simulink model "ieee_6_bus_base_case_hydro_dominated"  (R2015b)
settings: Solver=ode23t  StartTime=0.0  StopTime=25  FixedStep=Ts  RelTol=1e-3
values from neighbouring files (symbols this model uses):
  Cbase = 1/(100*pi*Xbase)    (= 1.34217357979e-05)    [ieee_6_bus.m]
  Lbase = Xbase/(100*pi)    (= 0.754903726073)    [ieee_6_bus.m]
  Ts = 1e-5    (= 1e-05)    [ieee_6_bus.m]
  Xbase = (Vbase^2)/Sbase    (= 237.16)    [ieee_6_bus.m]
undefined symbols (not defined in the file or in its folder): loadconnection, startup
libraries: powerlib x170, powerlib_meascontrol x15, simulink x10, sps_avr x4, powerlib_extras x1
(part 2 of 3)

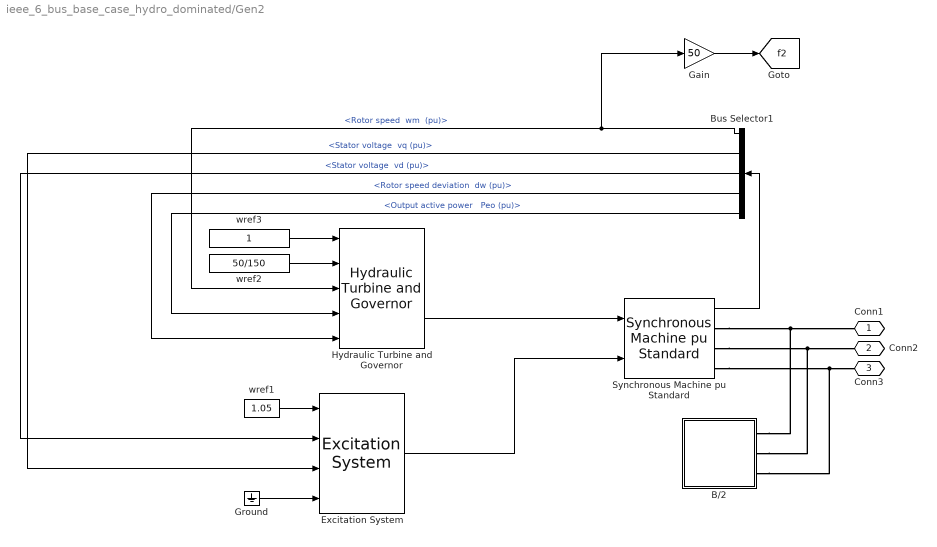
== system ieee_6_bus_base_case_hydro_dominated/Gen2 ==
  B/2 : Subsystem
  Bus Selector1 : BusSelector  OutputSignals="Mechanical.Rotor speed  wm  (pu),dq0 components.Stator voltage  vq (pu),dq0 components.Stator voltage  vd (pu),Mechanical.Rotor speed deviation  dw (pu),Output active power   Peo (pu)"
  Excitation System : sps_avr/Excitation System  tr=20e-3  reg=[ 350, 0.001 ]  exc=[ 1, 0 ]  tgr=[ 0, 0 ]  damp=[ 0.001, 0.1 ]  sat=[ 0, 0 ]  lim=[ -11.5, 11.5, 0 ]  v0="[1.0  1.28]"
  Gain : Gain  Gain=50
  Ground : Ground
  Hydraulic Turbine and Governor : powerlib/Machines/Hydraulic Turbine and Governor  sm="[ 10/3  0.07 ]"  gate="[  0.01  0.97518  -0.1  0.1 ]"  reg="[  0.05  1.163  0.105  0  0.01  ]"  hyd="[  0  2.67  ]"  dref=0  po=1/3
  Synchronous Machine pu Standard : powerlib/Machines/Synchronous Machine pu Standard  PresetModel=No  MechanicalLoad=Mechanical power Pm  ShowDetailedParameters=on  RotorType=Round  Units=per unit standard parameters  MeasurementBus=off  NominalParameters=[150e+06 690 50]  Reactances1=[ 1.81, 0.3, 0.23, 1.76, 0.65, 0.25, 0.15 ]  Reactances2=[2.24 0.17 0.12 1.02 0.13 0.08]  dAxisTimeConstants=Short-circuit  qAxisTimeConstants=Short-circuit  TimeConstants1="[ 4.4849  0.0681  0.1  ]"  TimeConstants2=[ 8.0, 0.03, 1.0, 0.07 ]  TimeConstants3="[  4.49  0.0681  0.0513  ]"  TimeConstants4=[ 8.0, 0.03, 0.3371, 0.0295 ]  TimeConstants5=[ 1.01, 0.053, 0.1 ]  TimeConstants6=[ 1.3201, 0.023, 1.0, 0.07 ]  TimeConstants7=[0.012 0.003 0.003]  TimeConstants8=[ 1.3201, 0.0231, 0.3371, 0.0295 ]  StatorResistance=0.00000107875  Mechanical=[4 0.02056 4]  PolePairs=20  InitialConditions="[ 0  0  0  0  0  0  0  0  1 ]"  SetSaturation=off  Saturation=[0.6404,0.7127,0.8441,0.9214,0.9956,1.082,1.19,1.316,1.457;0.7,0.7698,0.8872,0.9466,0.9969,1.046,1.1,1.151,1.201]  LoadFlowParameters=[1,0,0,0,0]  TsPowergui=0  TsBlock=-1  IterativeModel=Trapezoidal non iterative  BusType=PV  Pref=50e6  Qref=0  Qmin=-inf  Qmax=inf  PLF=0  QLF=0
  wref1 : Constant  Value=1.05
  wref2 : Constant  Value=50/150
  wref3 : Constant
  Conn1 : PMIOPort  Port=1  Side=Right
  Conn2 : PMIOPort  Port=2  Side=Right
  Conn3 : PMIOPort  Port=3  Side=Right
  tag scope: f2=global
  wires:
  Hydraulic Turbine and Governor/2 -> Synchronous Machine pu Standard/1
  Gain/1 -> [f2]
  Bus Selector1/2 -> Excitation System/3  "<Stator voltage  vq (pu)>"
  Bus Selector1/1 -> Hydraulic Turbine and Governor/3, Gain/1  "<Rotor speed  wm  (pu)>"
  Bus Selector1/3 -> Excitation System/2  "<Stator voltage  vd (pu)>"
  Excitation System/1 -> Synchronous Machine pu Standard/2
  Ground/1 -> Excitation System/4
  wref1/1 -> Excitation System/1
  Synchronous Machine pu Standard/1 -> Bus Selector1/1
  wref3/1 -> Hydraulic Turbine and Governor/1
  Bus Selector1/4 -> Hydraulic Turbine and Governor/5  "<Rotor speed deviation  dw (pu)>"
  Bus Selector1/5 -> Hydraulic Turbine and Governor/4  "<Output active power   Peo (pu)>"
  wref2/1 -> Hydraulic Turbine and Governor/2
  connections:
  Synchronous Machine pu Standard/RConn1 -- Conn1/RConn1 -- B/2/RConn1
  Synchronous Machine pu Standard/RConn2 -- Conn2/RConn1 -- B/2/RConn2
  Synchronous Machine pu Standard/RConn3 -- Conn3/RConn1 -- B/2/RConn3

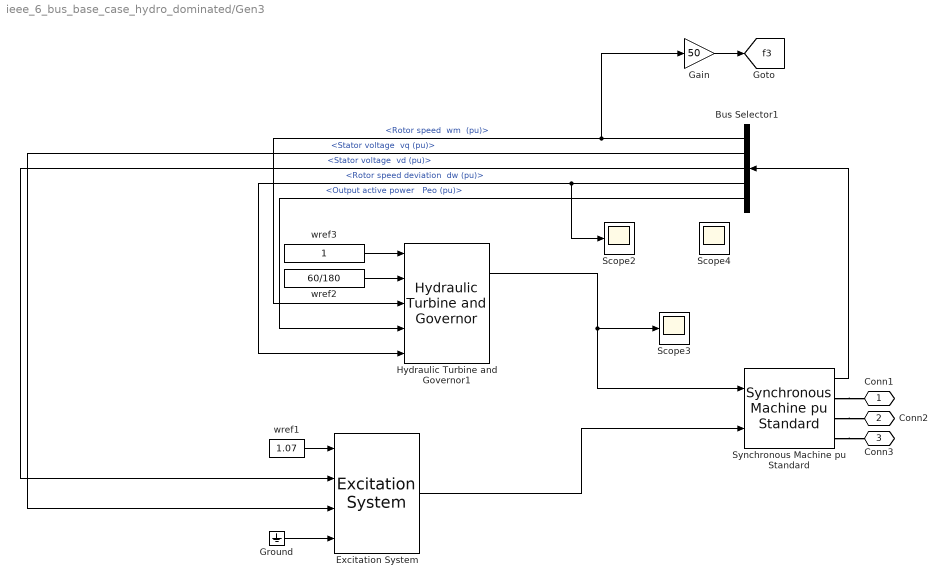
== system ieee_6_bus_base_case_hydro_dominated/Gen3 ==
  Bus Selector1 : BusSelector  OutputSignals="Mechanical.Rotor speed  wm  (pu),dq0 components.Stator voltage  vq (pu),dq0 components.Stator voltage  vd (pu),Mechanical.Rotor speed deviation  dw (pu),Output active power   Peo (pu)"
  Excitation System : sps_avr/Excitation System  tr=20e-3  reg=[ 350, 0.001 ]  exc=[ 1, 0 ]  tgr=[ 0, 0 ]  damp=[ 0.001, 0.1 ]  sat=[ 0, 0 ]  lim=[ -11.5, 11.5, 0 ]  v0="[1.0  1.28]"
  Gain : Gain  Gain=50
  Ground : Ground
  Hydraulic Turbine and Governor1 : powerlib/Machines/Hydraulic Turbine and Governor  sm="[ 10/3  0.07 ]"  gate="[  0.01  0.97518  -0.1  0.1 ]"  reg="[  0.05  1.163  0.105  0  0.01  ]"  hyd="[  0  2.67  ]"  dref=0  po=1/3
  Scope2 : Scope
  Scope3 : Scope
  Scope4 : Scope
  Synchronous Machine pu Standard : powerlib/Machines/Synchronous Machine pu Standard  PresetModel=No  MechanicalLoad=Mechanical power Pm  ShowDetailedParameters=on  RotorType=Round  Units=per unit standard parameters  MeasurementBus=off  NominalParameters=[180e+06 690 50]  Reactances1=[ 1.81, 0.3, 0.23, 1.76, 0.65, 0.25, 0.15 ]  Reactances2=[2.24 0.17 0.12 1.02 0.13 0.08]  dAxisTimeConstants=Short-circuit  qAxisTimeConstants=Short-circuit  TimeConstants1="[ 4.4849  0.0681  0.1  ]"  TimeConstants2=[ 8.0, 0.03, 1.0, 0.07 ]  TimeConstants3="[  4.49  0.0681  0.0513  ]"  TimeConstants4=[ 8.0, 0.03, 0.3371, 0.0295 ]  TimeConstants5=[ 1.01, 0.053, 0.1 ]  TimeConstants6=[ 1.3201, 0.023, 1.0, 0.07 ]  TimeConstants7=[0.012 0.003 0.003]  TimeConstants8=[ 1.3201, 0.0231, 0.3371, 0.0295 ]  StatorResistance=0.00000107875  Mechanical=[4 0.02056 4]  PolePairs=20  InitialConditions="[ 0  0  0  0  0  0  0  0  1 ]"  SetSaturation=off  Saturation=[0.6404,0.7127,0.8441,0.9214,0.9956,1.082,1.19,1.316,1.457;0.7,0.7698,0.8872,0.9466,0.9969,1.046,1.1,1.151,1.201]  LoadFlowParameters=[1,0,0,0,0]  TsPowergui=0  TsBlock=-1  IterativeModel=Trapezoidal non iterative  BusType=PV  Pref=60e6  Qref=0  Qmin=-inf  Qmax=inf  PLF=0  QLF=0
  wref1 : Constant  Value=1.07
  wref2 : Constant  Value=60/180
  wref3 : Constant
  Conn1 : PMIOPort  Port=1  Side=Right
  Conn2 : PMIOPort  Port=2  Side=Right
  Conn3 : PMIOPort  Port=3  Side=Right
  tag scope: f3=global
  wires:
  Synchronous Machine pu Standard/1 -> Bus Selector1/1
  wref1/1 -> Excitation System/1
  Ground/1 -> Excitation System/4
  Excitation System/1 -> Synchronous Machine pu Standard/2
  Bus Selector1/3 -> Excitation System/2  "<Stator voltage  vd (pu)>"
  Bus Selector1/1 -> Hydraulic Turbine and Governor1/3, Gain/1  "<Rotor speed  wm  (pu)>"
  Bus Selector1/2 -> Excitation System/3  "<Stator voltage  vq (pu)>"
  Gain/1 -> [f3]
  Hydraulic Turbine and Governor1/1 -> Synchronous Machine pu Standard/1, Scope3/1
  wref2/1 -> Hydraulic Turbine and Governor1/2
  wref3/1 -> Hydraulic Turbine and Governor1/1
  Bus Selector1/4 -> Hydraulic Turbine and Governor1/5, Scope2/1  "<Rotor speed deviation  dw (pu)>"
  Bus Selector1/5 -> Hydraulic Turbine and Governor1/4  "<Output active power   Peo (pu)>"
  connections:
  Synchronous Machine pu Standard/RConn3 -- Conn3/RConn1
  Synchronous Machine pu Standard/RConn2 -- Conn2/RConn1
  Synchronous Machine pu Standard/RConn1 -- Conn1/RConn1

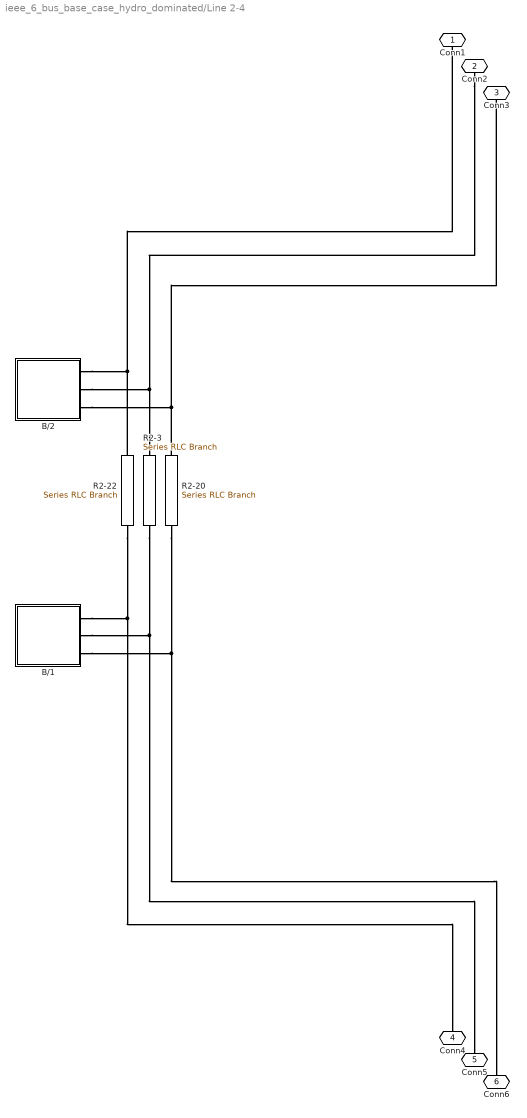
== system ieee_6_bus_base_case_hydro_dominated/Line 2-4 ==
  B/1 : Subsystem
  B/2 : Subsystem
  R2-20 : powerlib/Elements/Series RLC Branch  LConnTagsString=__new0  RConnTagsString=__new0  BranchType=RL  Resistance=0.05*Xbase  Inductance=0.1*Lbase  SetiL0=off  InitialCurrent=0  Capacitance=1e-6  Setx0=off  InitialVoltage=0  Measurements=None
  R2-22 : powerlib/Elements/Series RLC Branch  LConnTagsString=__new0  RConnTagsString=__new0  BranchType=RL  Resistance=0.05*Xbase  Inductance=0.1*Lbase  SetiL0=off  InitialCurrent=0  Capacitance=1e-6  Setx0=off  InitialVoltage=0  Measurements=None
  R2-3 : powerlib/Elements/Series RLC Branch  LConnTagsString=__new0  RConnTagsString=__new0  BranchType=RL  Resistance=0.05*Xbase  Inductance=0.1*Lbase  SetiL0=off  InitialCurrent=0  Capacitance=1e-6  Setx0=off  InitialVoltage=0  Measurements=None
  Conn1 : PMIOPort  Port=1  Side=Right
  Conn2 : PMIOPort  Port=2  Side=Right
  Conn3 : PMIOPort  Port=3  Side=Right
  Conn4 : PMIOPort  Port=4  Side=Left
  Conn5 : PMIOPort  Port=5  Side=Left
  Conn6 : PMIOPort  Port=6  Side=Left
  connections:
  R2-22/RConn1 -- B/1/RConn1 -- Conn4/RConn1
  R2-20/RConn1 -- B/1/RConn3 -- Conn6/RConn1
  Conn2/RConn1 -- B/2/RConn2 -- R2-3/LConn1
  R2-22/LConn1 -- B/2/RConn1 -- Conn1/RConn1
  R2-20/LConn1 -- B/2/RConn3 -- Conn3/RConn1
  R2-3/RConn1 -- B/1/RConn2 -- Conn5/RConn1

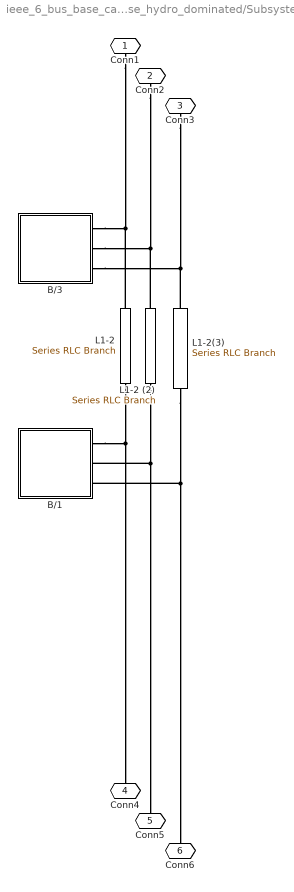
== system ieee_6_bus_base_case_hydro_dominated/Subsystem ==
  B/1 : Subsystem
  B/3 : Subsystem
  "L1-2 " : powerlib/Elements/Series RLC Branch  LConnTagsString=__new0  RConnTagsString=__new0  BranchType=RL  Resistance=0.1*Xbase  Inductance=0.2*Lbase  SetiL0=off  InitialCurrent=0  Capacitance=1e-6  Setx0=off  InitialVoltage=0  Measurements=None
  L1-2 (2) : powerlib/Elements/Series RLC Branch  LConnTagsString=__new0  RConnTagsString=__new0  BranchType=RL  Resistance=0.1*Xbase  Inductance=0.2*Lbase  SetiL0=off  InitialCurrent=0  Capacitance=1e-6  Setx0=off  InitialVoltage=0  Measurements=None
  L1-2(3) : powerlib/Elements/Series RLC Branch  LConnTagsString=__new0  RConnTagsString=__new0  BranchType=RL  Resistance=0.1*Xbase  Inductance=0.2*Lbase  SetiL0=off  InitialCurrent=0  Capacitance=1e-6  Setx0=off  InitialVoltage=0  Measurements=None
  Conn1 : PMIOPort  Port=1  Side=Right
  Conn2 : PMIOPort  Port=2  Side=Right
  Conn3 : PMIOPort  Port=3  Side=Right
  Conn4 : PMIOPort  Port=4  Side=Left
  Conn5 : PMIOPort  Port=5  Side=Left
  Conn6 : PMIOPort  Port=6  Side=Left
  connections:
  B/3/RConn1 -- Conn1/RConn1 -- "L1-2 "/LConn1
  L1-2 (2)/RConn1 -- Conn5/RConn1 -- B/1/RConn2
  "L1-2 "/RConn1 -- Conn4/RConn1 -- B/1/RConn1
  B/3/RConn3 -- Conn3/RConn1 -- L1-2(3)/LConn1
  L1-2(3)/RConn1 -- Conn6/RConn1 -- B/1/RConn3
  L1-2 (2)/LConn1 -- Conn2/RConn1 -- B/3/RConn2

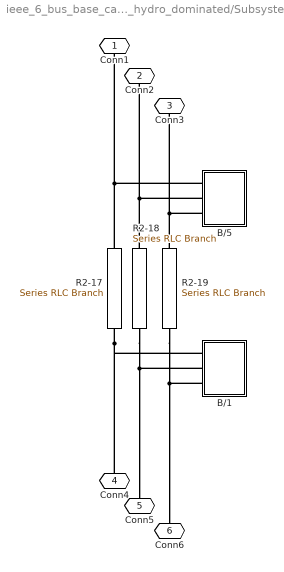
== system ieee_6_bus_base_case_hydro_dominated/Subsystem1 ==
  B/1 : Subsystem
  B/5 : Subsystem
  R2-17 : powerlib/Elements/Series RLC Branch  LConnTagsString=__new0  RConnTagsString=__new0  BranchType=RL  Resistance=0.05*Xbase  Inductance=0.2*Lbase  SetiL0=off  InitialCurrent=0  Capacitance=1e-6  Setx0=off  InitialVoltage=0  Measurements=None
  R2-18 : powerlib/Elements/Series RLC Branch  LConnTagsString=__new0  RConnTagsString=__new0  BranchType=RL  Resistance=0.05*Xbase  Inductance=0.2*Lbase  SetiL0=off  InitialCurrent=0  Capacitance=1e-6  Setx0=off  InitialVoltage=0  Measurements=None
  R2-19 : powerlib/Elements/Series RLC Branch  LConnTagsString=__new0  RConnTagsString=__new0  BranchType=RL  Resistance=0.05*Xbase  Inductance=0.2*Lbase  SetiL0=off  InitialCurrent=0  Capacitance=1e-6  Setx0=off  InitialVoltage=0  Measurements=None
  Conn1 : PMIOPort  Port=1  Side=Right
  Conn2 : PMIOPort  Port=2  Side=Right
  Conn3 : PMIOPort  Port=3  Side=Right
  Conn4 : PMIOPort  Port=4  Side=Left
  Conn5 : PMIOPort  Port=5  Side=Left
  Conn6 : PMIOPort  Port=6  Side=Left
  connections:
  R2-18/RConn1 -- Conn5/RConn1 -- B/1/RConn2
  R2-19/RConn1 -- Conn6/RConn1 -- B/1/RConn3
  R2-17/RConn1 -- Conn4/RConn1 -- B/1/RConn1
  B/5/RConn1 -- Conn1/RConn1 -- R2-17/LConn1
  R2-18/LConn1 -- Conn2/RConn1 -- B/5/RConn2
  R2-19/LConn1 -- Conn3/RConn1 -- B/5/RConn3

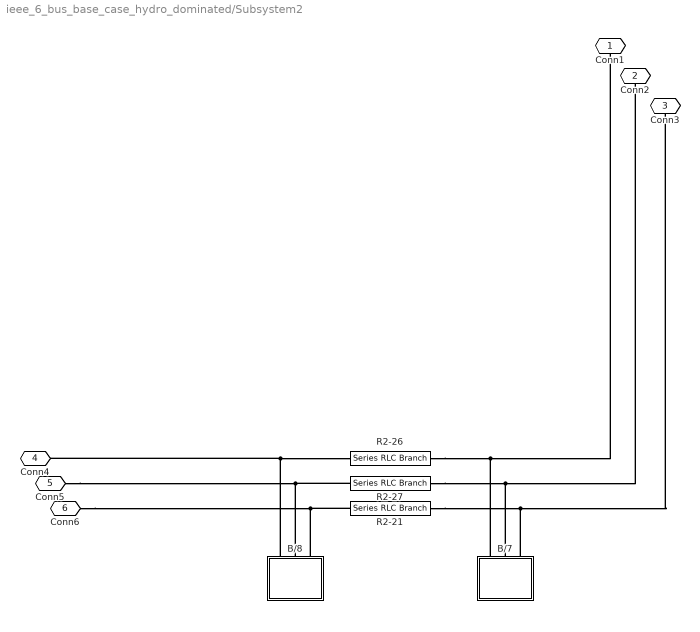
== system ieee_6_bus_base_case_hydro_dominated/Subsystem2 ==
  B/7 : Subsystem
  B/8 : Subsystem
  R2-21 : powerlib/Elements/Series RLC Branch  LConnTagsString=__new0  RConnTagsString=__new0  BranchType=RL  Resistance=0.2*Xbase  Inductance=0.4*Lbase  SetiL0=off  InitialCurrent=0  Capacitance=1e-6  Setx0=off  InitialVoltage=0  Measurements=None
  R2-26 : powerlib/Elements/Series RLC Branch  LConnTagsString=__new0  RConnTagsString=__new0  BranchType=RL  Resistance=0.2*Xbase  Inductance=0.4*Lbase  SetiL0=off  InitialCurrent=0  Capacitance=1e-6  Setx0=off  InitialVoltage=0  Measurements=None
  R2-27 : powerlib/Elements/Series RLC Branch  LConnTagsString=__new0  RConnTagsString=__new0  BranchType=RL  Resistance=0.2*Xbase  Inductance=0.4*Lbase  SetiL0=off  InitialCurrent=0  Capacitance=1e-6  Setx0=off  InitialVoltage=0  Measurements=None
  Conn1 : PMIOPort  Port=1  Side=Right
  Conn2 : PMIOPort  Port=2  Side=Right
  Conn3 : PMIOPort  Port=3  Side=Right
  Conn4 : PMIOPort  Port=4  Side=Left
  Conn5 : PMIOPort  Port=5  Side=Left
  Conn6 : PMIOPort  Port=6  Side=Left
  connections:
  B/8/RConn3 -- Conn6/RConn1 -- R2-21/RConn1
  B/8/RConn1 -- Conn4/RConn1 -- R2-26/RConn1
  R2-27/RConn1 -- Conn5/RConn1 -- B/8/RConn2
  B/7/RConn1 -- Conn1/RConn1 -- R2-26/LConn1
  B/7/RConn2 -- Conn2/RConn1 -- R2-27/LConn1
  B/7/RConn3 -- Conn3/RConn1 -- R2-21/LConn1

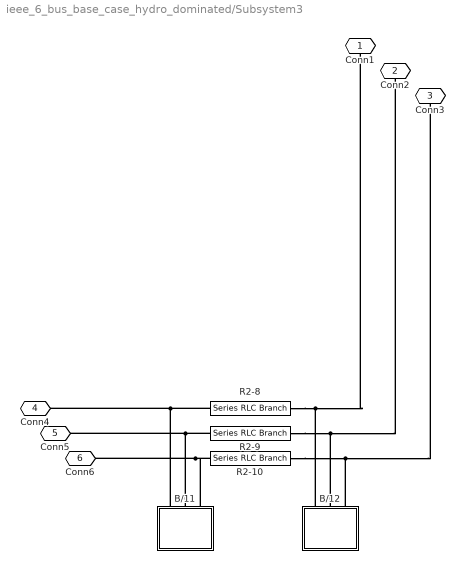
== system ieee_6_bus_base_case_hydro_dominated/Subsystem3 ==
  B/11 : Subsystem
  B/12 : Subsystem
  R2-10 : powerlib/Elements/Series RLC Branch  LConnTagsString=__new0  RConnTagsString=__new0  BranchType=RL  Resistance=0.1*Xbase  Inductance=0.3*Lbase  SetiL0=off  InitialCurrent=0  Capacitance=1e-6  Setx0=off  InitialVoltage=0  Measurements=None
  R2-8 : powerlib/Elements/Series RLC Branch  LConnTagsString=__new0  RConnTagsString=__new0  BranchType=RL  Resistance=0.1*Xbase  Inductance=0.3*Lbase  SetiL0=off  InitialCurrent=0  Capacitance=1e-6  Setx0=off  InitialVoltage=0  Measurements=None
  R2-9 : powerlib/Elements/Series RLC Branch  LConnTagsString=__new0  RConnTagsString=__new0  BranchType=RL  Resistance=0.1*Xbase  Inductance=0.3*Lbase  SetiL0=off  InitialCurrent=0  Capacitance=1e-6  Setx0=off  InitialVoltage=0  Measurements=None
  Conn1 : PMIOPort  Port=1  Side=Right
  Conn2 : PMIOPort  Port=2  Side=Right
  Conn3 : PMIOPort  Port=3  Side=Right
  Conn4 : PMIOPort  Port=4  Side=Left
  Conn5 : PMIOPort  Port=5  Side=Left
  Conn6 : PMIOPort  Port=6  Side=Left
  connections:
  R2-10/RConn1 -- Conn3/RConn1 -- B/12/RConn3
  R2-10/LConn1 -- Conn6/RConn1 -- B/11/RConn3
  R2-9/RConn1 -- Conn2/RConn1 -- B/12/RConn2
  B/12/RConn1 -- Conn1/RConn1 -- R2-8/RConn1
  R2-9/LConn1 -- Conn5/RConn1 -- B/11/RConn2
  R2-8/LConn1 -- Conn4/RConn1 -- B/11/RConn1

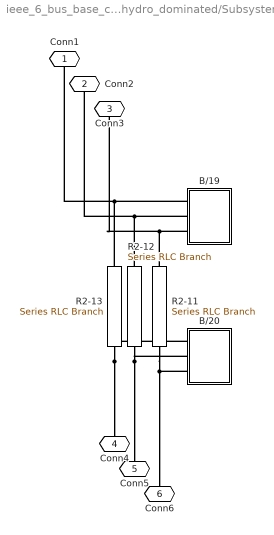
== system ieee_6_bus_base_case_hydro_dominated/Subsystem4 ==
  B/19 : Subsystem
  B/20 : Subsystem
  R2-11 : powerlib/Elements/Series RLC Branch  LConnTagsString=__new0  RConnTagsString=__new0  BranchType=RL  Resistance=0.12*Xbase  Inductance=0.26*Lbase  SetiL0=off  InitialCurrent=0  Capacitance=1e-6  Setx0=off  InitialVoltage=0  Measurements=None
  R2-12 : powerlib/Elements/Series RLC Branch  LConnTagsString=__new0  RConnTagsString=__new0  BranchType=RL  Resistance=0.12*Xbase  Inductance=0.26*Lbase  SetiL0=off  InitialCurrent=0  Capacitance=1e-6  Setx0=off  InitialVoltage=0  Measurements=None
  R2-13 : powerlib/Elements/Series RLC Branch  LConnTagsString=__new0  RConnTagsString=__new0  BranchType=RL  Resistance=0.12*Xbase  Inductance=0.26*Lbase  SetiL0=off  InitialCurrent=0  Capacitance=1e-6  Setx0=off  InitialVoltage=0  Measurements=None
  Conn1 : PMIOPort  Port=1  Side=Right
  Conn2 : PMIOPort  Port=2  Side=Right
  Conn3 : PMIOPort  Port=3  Side=Right
  Conn4 : PMIOPort  Port=4  Side=Left
  Conn5 : PMIOPort  Port=5  Side=Left
  Conn6 : PMIOPort  Port=6  Side=Left
  connections:
  R2-12/LConn1 -- Conn2/RConn1 -- B/19/RConn2
  B/20/RConn1 -- Conn4/RConn1 -- R2-13/RConn1
  B/20/RConn3 -- Conn6/RConn1 -- R2-11/RConn1
  B/19/RConn1 -- Conn1/RConn1 -- R2-13/LConn1
  B/19/RConn3 -- Conn3/RConn1 -- R2-11/LConn1
  B/20/RConn2 -- Conn5/RConn1 -- R2-12/RConn1

== system ieee_6_bus_base_case_hydro_dominated/Subsystem5 ==
  B/10 : Subsystem
  B/9 : Subsystem
  R2-4 : powerlib/Elements/Series RLC Branch  LConnTagsString=__new0  RConnTagsString=__new0  BranchType=RL  Resistance=0.02*Xbase  Inductance=0.1*Lbase  SetiL0=off  InitialCurrent=0  Capacitance=1e-6  Setx0=off  InitialVoltage=0  Measurements=None
  R2-5 : powerlib/Elements/Series RLC Branch  LConnTagsString=__new0  RConnTagsString=__new0  BranchType=RL  Resistance=0.02*Xbase  Inductance=0.1*Lbase  SetiL0=off  InitialCurrent=0  Capacitance=1e-6  Setx0=off  InitialVoltage=0  Measurements=None
  R2-7 : powerlib/Elements/Series RLC Branch  LConnTagsString=__new0  RConnTagsString=__new0  BranchType=RL  Resistance=0.02*Xbase  Inductance=0.1*Lbase  SetiL0=off  InitialCurrent=0  Capacitance=1e-6  Setx0=off  InitialVoltage=0  Measurements=None
  Conn1 : PMIOPort  Port=1  Side=Left
  Conn2 : PMIOPort  Port=2  Side=Right
  Conn3 : PMIOPort  Port=3  Side=Left
  Conn4 : PMIOPort  Port=4  Side=Right
  Conn5 : PMIOPort  Port=5  Side=Left
  Conn6 : PMIOPort  Port=6  Side=Right
  connections:
  R2-4/LConn1 -- Conn1/RConn1 -- B/9/RConn1
  B/9/RConn3 -- Conn5/RConn1 -- R2-7/LConn1
  R2-5/LConn1 -- Conn3/RConn1 -- B/9/RConn2
  B/10/RConn1 -- Conn2/RConn1 -- R2-4/RConn1
  R2-7/RConn1 -- Conn6/RConn1 -- B/10/RConn3
  B/10/RConn2 -- Conn4/RConn1 -- R2-5/RConn1

== system ieee_6_bus_base_case_hydro_dominated/Subsystem6 ==
  B/16 : Subsystem
  B/18 : Subsystem
  R2-23 : powerlib/Elements/Series RLC Branch  LConnTagsString=__new0  RConnTagsString=__new0  BranchType=RL  Resistance=0.1*Xbase  Inductance=0.3*Lbase  SetiL0=off  InitialCurrent=0  Capacitance=1e-6  Setx0=off  InitialVoltage=0  Measurements=None
  R2-25 : powerlib/Elements/Series RLC Branch  LConnTagsString=__new0  RConnTagsString=__new0  BranchType=RL  Resistance=0.1*Xbase  Inductance=0.3*Lbase  SetiL0=off  InitialCurrent=0  Capacitance=1e-6  Setx0=off  InitialVoltage=0  Measurements=None
  R2-29 : powerlib/Elements/Series RLC Branch  LConnTagsString=__new0  RConnTagsString=__new0  BranchType=RL  Resistance=0.1*Xbase  Inductance=0.3*Lbase  SetiL0=off  InitialCurrent=0  Capacitance=1e-6  Setx0=off  InitialVoltage=0  Measurements=None
  Conn1 : PMIOPort  Port=1  Side=Right
  Conn2 : PMIOPort  Port=2  Side=Right
  Conn3 : PMIOPort  Port=3  Side=Right
  Conn4 : PMIOPort  Port=4  Side=Left
  Conn5 : PMIOPort  Port=5  Side=Left
  Conn6 : PMIOPort  Port=6  Side=Left
  connections:
  R2-25/LConn1 -- Conn3/RConn1 -- B/16/RConn3
  R2-23/LConn1 -- Conn2/RConn1 -- B/16/RConn2
  B/18/RConn2 -- Conn5/RConn1 -- R2-23/RConn1
  B/18/RConn3 -- Conn6/RConn1 -- R2-25/RConn1
  R2-29/LConn1 -- Conn1/RConn1 -- B/16/RConn1
  B/18/RConn1 -- Conn4/RConn1 -- R2-29/RConn1

== system ieee_6_bus_base_case_hydro_dominated/Subsystem7 ==
  B/13 : Subsystem
  B/14 : Subsystem
  R2-28 : powerlib/Elements/Series RLC Branch  LConnTagsString=__new0  RConnTagsString=__new0  BranchType=RL  Resistance=0.07*Xbase  Inductance=0.2*Lbase  SetiL0=off  InitialCurrent=0  Capacitance=1e-6  Setx0=off  InitialVoltage=0  Measurements=None
  R2-30 : powerlib/Elements/Series RLC Branch  LConnTagsString=__new0  RConnTagsString=__new0  BranchType=RL  Resistance=0.07*Xbase  Inductance=0.2*Lbase  SetiL0=off  InitialCurrent=0  Capacitance=1e-6  Setx0=off  InitialVoltage=0  Measurements=None
  R2-6 : powerlib/Elements/Series RLC Branch  LConnTagsString=__new0  RConnTagsString=__new0  BranchType=RL  Resistance=0.07*Xbase  Inductance=0.2*Lbase  SetiL0=off  InitialCurrent=0  Capacitance=1e-6  Setx0=off  InitialVoltage=0  Measurements=None
  Conn1 : PMIOPort  Port=1  Side=Left
  Conn2 : PMIOPort  Port=2  Side=Right
  Conn3 : PMIOPort  Port=3  Side=Left
  Conn4 : PMIOPort  Port=4  Side=Right
  Conn5 : PMIOPort  Port=5  Side=Left
  Conn6 : PMIOPort  Port=6  Side=Right
  connections:
  B/14/RConn3 -- Conn5/RConn1 -- R2-30/LConn1
  B/14/RConn2 -- Conn3/RConn1 -- R2-28/LConn1
  R2-6/LConn1 -- Conn1/RConn1 -- B/14/RConn1
  R2-6/RConn1 -- Conn2/RConn1 -- B/13/RConn1
  B/13/RConn2 -- Conn4/RConn1 -- R2-28/RConn1
  R2-30/RConn1 -- Conn6/RConn1 -- B/13/RConn3

== system ieee_6_bus_base_case_hydro_dominated/Subsystem8 ==
  B/21 : Subsystem
  B/22 : Subsystem
  R2-1 : powerlib/Elements/Series RLC Branch  LConnTagsString=__new0  RConnTagsString=__new0  BranchType=RL  Resistance=0.05*Xbase  Inductance=0.25*Lbase  SetiL0=off  InitialCurrent=0  Capacitance=1e-6  Setx0=off  InitialVoltage=0  Measurements=None
  R2-2 : powerlib/Elements/Series RLC Branch  LConnTagsString=__new0  RConnTagsString=__new0  BranchType=RL  Resistance=0.05*Xbase  Inductance=0.25*Lbase  SetiL0=off  InitialCurrent=0  Capacitance=1e-6  Setx0=off  InitialVoltage=0  Measurements=None
  R2-24 : powerlib/Elements/Series RLC Branch  LConnTagsString=__new0  RConnTagsString=__new0  BranchType=RL  Resistance=0.05*Xbase  Inductance=0.25*Lbase  SetiL0=off  InitialCurrent=0  Capacitance=1e-6  Setx0=off  InitialVoltage=0  Measurements=None
  Conn1 : PMIOPort  Port=1  Side=Right
  Conn2 : PMIOPort  Port=2  Side=Right
  Conn3 : PMIOPort  Port=3  Side=Right
  Conn4 : PMIOPort  Port=4  Side=Left
  Conn5 : PMIOPort  Port=5  Side=Left
  Conn6 : PMIOPort  Port=6  Side=Left
  connections:
  B/21/RConn1 -- R2-24/LConn1 -- Conn1/RConn1
  R2-2/RConn1 -- Conn6/RConn1 -- B/22/RConn3
  B/22/RConn1 -- Conn4/RConn1 -- R2-24/RConn1
  B/21/RConn2 -- R2-1/LConn1 -- Conn2/RConn1
  B/21/RConn3 -- R2-2/LConn1 -- Conn3/RConn1
  R2-1/RConn1 -- Conn5/RConn1 -- B/22/RConn2

== system ieee_6_bus_base_case_hydro_dominated/Subsystem9 ==
  B/15 : Subsystem
  B/6 : Subsystem
  R2-14 : powerlib/Elements/Series RLC Branch  LConnTagsString=__new0  RConnTagsString=__new0  BranchType=RL  Resistance=0.08*Xbase  Inductance=0.3*Xbase  SetiL0=off  InitialCurrent=0  Capacitance=1e-6  Setx0=off  InitialVoltage=0  Measurements=None
  R2-15 : powerlib/Elements/Series RLC Branch  LConnTagsString=__new0  RConnTagsString=__new0  BranchType=RL  Resistance=0.08*Xbase  Inductance=0.3*Xbase  SetiL0=off  InitialCurrent=0  Capacitance=1e-6  Setx0=off  InitialVoltage=0  Measurements=None
  R2-16 : powerlib/Elements/Series RLC Branch  LConnTagsString=__new0  RConnTagsString=__new0  BranchType=RL  Resistance=0.08*Xbase  Inductance=0.3*Xbase  SetiL0=off  InitialCurrent=0  Capacitance=1e-6  Setx0=off  InitialVoltage=0  Measurements=None
  Conn1 : PMIOPort  Port=1  Side=Left
  Conn2 : PMIOPort  Port=2  Side=Right
  Conn3 : PMIOPort  Port=3  Side=Left
  Conn4 : PMIOPort  Port=4  Side=Right
  Conn5 : PMIOPort  Port=5  Side=Left
  Conn6 : PMIOPort  Port=6  Side=Right
  connections:
  R2-15/LConn1 -- Conn3/RConn1 -- B/15/RConn2
  B/6/RConn2 -- Conn4/RConn1 -- R2-15/RConn1
  B/6/RConn1 -- Conn2/RConn1 -- R2-14/RConn1
  B/6/RConn3 -- Conn6/RConn1 -- R2-16/RConn1
  B/15/RConn3 -- Conn5/RConn1 -- R2-16/LConn1
  B/15/RConn1 -- Conn1/RConn1 -- R2-14/LConn1

== system ieee_6_bus_base_case_hydro_dominated/GE2.75 - 3/Gearbox ==
  Tt : Inport
  Divide : Product  Inputs=*/
  Gear Ratio1 : Constant  Value=gear
  Tt' : Outport
  wires:
  Divide/1 -> Tt'/1
  Tt/1 -> Divide/1
  Gear Ratio1/1 -> Divide/2

== system ieee_6_bus_base_case_hydro_dominated/GE2.75 - 3/Subsystem ==
  In1 : Inport
  Enable : EnablePort
  Out1 : Outport
  wires:
  In1/1 -> Out1/1

== system ieee_6_bus_base_case_hydro_dominated/GE2.75 - 3/Subsystem1 ==
  In1 : Inport
  Enable : EnablePort
  Out1 : Outport
  wires:
  In1/1 -> Out1/1

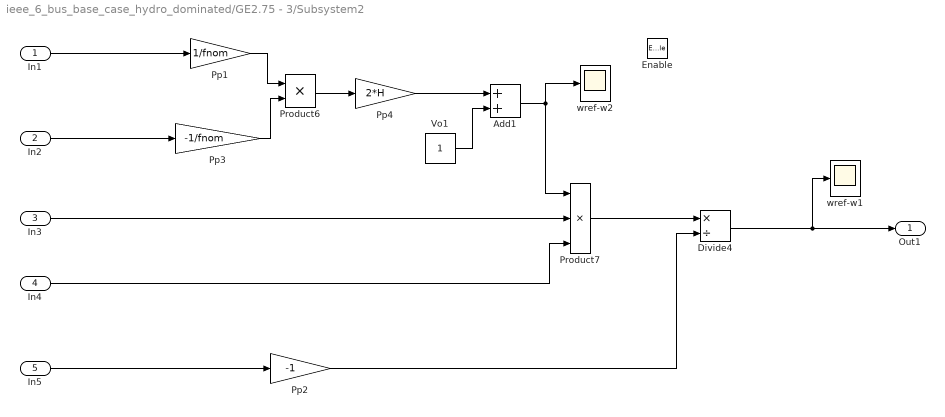
== system ieee_6_bus_base_case_hydro_dominated/GE2.75 - 3/Subsystem2 ==
  In1 : Inport
  In2 : Inport  Port=2
  In3 : Inport  Port=3
  In4 : Inport  Port=4
  In5 : Inport  Port=5
  Enable : EnablePort
  Add1 : Sum
  Divide4 : Product  Inputs=*/
  Pp1 : Gain  Gain=1/fnom
  Pp2 : Gain  Gain=-1
  Pp3 : Gain  Gain=-1/fnom
  Pp4 : Gain  Gain=2*H
  Product6 : Product
  Product7 : Product  Inputs=3
  Vo1 : Constant
  wref-w1 : Scope
  wref-w2 : Scope
  Out1 : Outport
  wires:
  Pp2/1 -> Divide4/2
  Pp4/1 -> Add1/1
  In1/1 -> Pp1/1
  Divide4/1 -> Out1/1, wref-w1/1
  In4/1 -> Product7/3
  Product7/1 -> Divide4/1
  Product6/1 -> Pp4/1
  Add1/1 -> wref-w2/1, Product7/1
  Vo1/1 -> Add1/2
  Pp1/1 -> Product6/1
  In5/1 -> Pp2/1
  In3/1 -> Product7/2
  In2/1 -> Pp3/1
  Pp3/1 -> Product6/2

== system ieee_6_bus_base_case_hydro_dominated/GE2.75 - 3/pitch angle controller ==
  wr : Inport
  Constant1 : Constant  Value=1735/1500  SampleTime=Ts
  pitch angle controller : Subsystem
  Beta : Outport
  wires:
  wr/1 -> pitch angle controller/1(wg)
  pitch angle controller/1(pitch) -> Beta/1
  Constant1/1 -> pitch angle controller/2(Ref)

== system ieee_6_bus_base_case_hydro_dominated/Gen2/B//2 ==
  R2-1 : powerlib/Elements/Series RLC Branch  LConnTagsString=__new0  RConnTagsString=__new0  BranchType=R  Resistance=10000000000  Inductance=1e-3  SetiL0=off  InitialCurrent=0  Capacitance=1000000*Cbase  Setx0=off  InitialVoltage=0  Measurements=None
  R2-2 : powerlib/Elements/Series RLC Branch  LConnTagsString=__new0  RConnTagsString=__new0  BranchType=R  Resistance=10000000000  Inductance=1e-3  SetiL0=off  InitialCurrent=0  Capacitance=1000000*Cbase  Setx0=off  InitialVoltage=0  Measurements=None
  R2-32 : powerlib/Elements/Series RLC Branch  LConnTagsString=__new0  RConnTagsString=__new0  BranchType=R  Resistance=10000000000  Inductance=1e-3  SetiL0=off  InitialCurrent=0  Capacitance=1000000*Cbase  Setx0=off  InitialVoltage=0  Measurements=None
  Conn1 : PMIOPort  Port=1  Side=Right
  Conn2 : PMIOPort  Port=2  Side=Right
  Conn3 : PMIOPort  Port=3  Side=Right
  connections:
  R2-1/LConn1 -- Conn2/RConn1
  R2-1/RConn1 -- R2-32/RConn1 -- R2-2/RConn1
  R2-32/LConn1 -- Conn1/RConn1
  R2-2/LConn1 -- Conn3/RConn1

== system ieee_6_bus_base_case_hydro_dominated/Line 2-4/B//1 ==
  Ground : powerlib/Elements/Ground  LConnTagsString=a
  R2-1 : powerlib/Elements/Series RLC Branch  LConnTagsString=__new0  RConnTagsString=__new0  BranchType=C  Resistance=1  Inductance=1e-3  SetiL0=off  InitialCurrent=0  Capacitance=Cbase/50  Setx0=off  InitialVoltage=0  Measurements=None
  R2-2 : powerlib/Elements/Series RLC Branch  LConnTagsString=__new0  RConnTagsString=__new0  BranchType=C  Resistance=1  Inductance=1e-3  SetiL0=off  InitialCurrent=0  Capacitance=Cbase/50  Setx0=off  InitialVoltage=0  Measurements=None
  R2-32 : powerlib/Elements/Series RLC Branch  LConnTagsString=__new0  RConnTagsString=__new0  BranchType=C  Resistance=1  Inductance=1e-3  SetiL0=off  InitialCurrent=0  Capacitance=Cbase/50  Setx0=off  InitialVoltage=0  Measurements=None
  Conn1 : PMIOPort  Port=1  Side=Right
  Conn2 : PMIOPort  Port=2  Side=Right
  Conn3 : PMIOPort  Port=3  Side=Right
  connections:
  R2-32/LConn1 -- Conn1/RConn1
  R2-2/RConn1 -- R2-32/RConn1 -- Ground/LConn1 -- R2-1/RConn1
  R2-2/LConn1 -- Conn3/RConn1
  R2-1/LConn1 -- Conn2/RConn1

== system ieee_6_bus_base_case_hydro_dominated/Line 2-4/B//2 ==
  Ground : powerlib/Elements/Ground  LConnTagsString=a
  R2-1 : powerlib/Elements/Series RLC Branch  LConnTagsString=__new0  RConnTagsString=__new0  BranchType=C  Resistance=1  Inductance=1e-3  SetiL0=off  InitialCurrent=0  Capacitance=Cbase/50  Setx0=off  InitialVoltage=0  Measurements=None
  R2-2 : powerlib/Elements/Series RLC Branch  LConnTagsString=__new0  RConnTagsString=__new0  BranchType=C  Resistance=1  Inductance=1e-3  SetiL0=off  InitialCurrent=0  Capacitance=Cbase/50  Setx0=off  InitialVoltage=0  Measurements=None
  R2-32 : powerlib/Elements/Series RLC Branch  LConnTagsString=__new0  RConnTagsString=__new0  BranchType=C  Resistance=1  Inductance=1e-3  SetiL0=off  InitialCurrent=0  Capacitance=Cbase/50  Setx0=off  InitialVoltage=0  Measurements=None
  Conn1 : PMIOPort  Port=1  Side=Right
  Conn2 : PMIOPort  Port=2  Side=Right
  Conn3 : PMIOPort  Port=3  Side=Right
  connections:
  R2-1/LConn1 -- Conn2/RConn1
  R2-2/LConn1 -- Conn3/RConn1
  Ground/LConn1 -- R2-2/RConn1 -- R2-1/RConn1 -- R2-32/RConn1
  R2-32/LConn1 -- Conn1/RConn1

== system ieee_6_bus_base_case_hydro_dominated/Subsystem/B//1 ==
  C1 : powerlib/Elements/Series RLC Branch  LConnTagsString=__new0  RConnTagsString=__new0  BranchType=C  Resistance=1  Inductance=1e-3  SetiL0=off  InitialCurrent=0  Capacitance=Cbase/25  Setx0=off  InitialVoltage=0  Measurements=None
  C2 : powerlib/Elements/Series RLC Branch  LConnTagsString=__new0  RConnTagsString=__new0  BranchType=C  Resistance=1  Inductance=1e-3  SetiL0=off  InitialCurrent=0  Capacitance=Cbase/25  Setx0=off  InitialVoltage=0  Measurements=None
  C3 : powerlib/Elements/Series RLC Branch  LConnTagsString=__new0  RConnTagsString=__new0  BranchType=C  Resistance=1  Inductance=1e-3  SetiL0=off  InitialCurrent=0  Capacitance=Cbase/25  Setx0=off  InitialVoltage=0  Measurements=None
  Ground : powerlib/Elements/Ground  LConnTagsString=a
  Conn1 : PMIOPort  Port=1  Side=Right
  Conn2 : PMIOPort  Port=2  Side=Right
  Conn3 : PMIOPort  Port=3  Side=Right
  connections:
  C1/LConn1 -- Conn1/RConn1
  C3/RConn1 -- Ground/LConn1 -- C1/RConn1 -- C2/RConn1
  C3/LConn1 -- Conn3/RConn1
  C2/LConn1 -- Conn2/RConn1

== system ieee_6_bus_base_case_hydro_dominated/Subsystem/B//3 ==
  C1 : powerlib/Elements/Series RLC Branch  LConnTagsString=__new0  RConnTagsString=__new0  BranchType=C  Resistance=1  Inductance=1e-3  SetiL0=off  InitialCurrent=0  Capacitance=Cbase/25  Setx0=off  InitialVoltage=0  Measurements=None
  C2 : powerlib/Elements/Series RLC Branch  LConnTagsString=__new0  RConnTagsString=__new0  BranchType=C  Resistance=1  Inductance=1e-3  SetiL0=off  InitialCurrent=0  Capacitance=Cbase/25  Setx0=off  InitialVoltage=0  Measurements=None
  C3 : powerlib/Elements/Series RLC Branch  LConnTagsString=__new0  RConnTagsString=__new0  BranchType=C  Resistance=1  Inductance=1e-3  SetiL0=off  InitialCurrent=0  Capacitance=Cbase/25  Setx0=off  InitialVoltage=0  Measurements=None
  Ground : powerlib/Elements/Ground  LConnTagsString=a
  Conn1 : PMIOPort  Port=1  Side=Right
  Conn2 : PMIOPort  Port=2  Side=Right
  Conn3 : PMIOPort  Port=3  Side=Right
  connections:
  C2/LConn1 -- Conn2/RConn1
  C3/LConn1 -- Conn3/RConn1
  C1/RConn1 -- C3/RConn1 -- C2/RConn1 -- Ground/LConn1
  C1/LConn1 -- Conn1/RConn1

== system ieee_6_bus_base_case_hydro_dominated/Subsystem1/B//1 ==
  Ground : powerlib/Elements/Ground  LConnTagsString=a
  R2-1 : powerlib/Elements/Series RLC Branch  LConnTagsString=__new0  RConnTagsString=__new0  BranchType=C  Resistance=1  Inductance=1e-3  SetiL0=off  InitialCurrent=0  Capacitance=Cbase/25  Setx0=off  InitialVoltage=0  Measurements=None
  R2-2 : powerlib/Elements/Series RLC Branch  LConnTagsString=__new0  RConnTagsString=__new0  BranchType=C  Resistance=1  Inductance=1e-3  SetiL0=off  InitialCurrent=0  Capacitance=Cbase/25  Setx0=off  InitialVoltage=0  Measurements=None
  R2-32 : powerlib/Elements/Series RLC Branch  LConnTagsString=__new0  RConnTagsString=__new0  BranchType=C  Resistance=1  Inductance=1e-3  SetiL0=off  InitialCurrent=0  Capacitance=Cbase/25  Setx0=off  InitialVoltage=0  Measurements=None
  Conn1 : PMIOPort  Port=1  Side=Right
  Conn2 : PMIOPort  Port=2  Side=Right
  Conn3 : PMIOPort  Port=3  Side=Right
  connections:
  R2-32/LConn1 -- Conn1/RConn1
  R2-2/RConn1 -- Ground/LConn1 -- R2-32/RConn1 -- R2-1/RConn1
  R2-2/LConn1 -- Conn3/RConn1
  R2-1/LConn1 -- Conn2/RConn1

== system ieee_6_bus_base_case_hydro_dominated/Subsystem1/B//5 ==
  Ground : powerlib/Elements/Ground  LConnTagsString=a
  R2-1 : powerlib/Elements/Series RLC Branch  LConnTagsString=__new0  RConnTagsString=__new0  BranchType=C  Resistance=1  Inductance=1e-3  SetiL0=off  InitialCurrent=0  Capacitance=Cbase/25  Setx0=off  InitialVoltage=0  Measurements=None
  R2-2 : powerlib/Elements/Series RLC Branch  LConnTagsString=__new0  RConnTagsString=__new0  BranchType=C  Resistance=1  Inductance=1e-3  SetiL0=off  InitialCurrent=0  Capacitance=Cbase/25  Setx0=off  InitialVoltage=0  Measurements=None
  R2-32 : powerlib/Elements/Series RLC Branch  LConnTagsString=__new0  RConnTagsString=__new0  BranchType=C  Resistance=1  Inductance=1e-3  SetiL0=off  InitialCurrent=0  Capacitance=Cbase/25  Setx0=off  InitialVoltage=0  Measurements=None
  Conn1 : PMIOPort  Port=1  Side=Right
  Conn2 : PMIOPort  Port=2  Side=Right
  Conn3 : PMIOPort  Port=3  Side=Right
  connections:
  R2-1/LConn1 -- Conn2/RConn1
  R2-2/LConn1 -- Conn3/RConn1
  R2-32/RConn1 -- R2-2/RConn1 -- R2-1/RConn1 -- Ground/LConn1
  R2-32/LConn1 -- Conn1/RConn1

== system ieee_6_bus_base_case_hydro_dominated/Subsystem2/B//7 ==
  Ground : powerlib/Elements/Ground  LConnTagsString=a
  R2-1 : powerlib/Elements/Series RLC Branch  LConnTagsString=__new0  RConnTagsString=__new0  BranchType=C  Resistance=1  Inductance=1e-3  SetiL0=off  InitialCurrent=0  Capacitance=Cbase/12.5  Setx0=off  InitialVoltage=0  Measurements=None
  R2-2 : powerlib/Elements/Series RLC Branch  LConnTagsString=__new0  RConnTagsString=__new0  BranchType=C  Resistance=1  Inductance=1e-3  SetiL0=off  InitialCurrent=0  Capacitance=Cbase/12.5  Setx0=off  InitialVoltage=0  Measurements=None
  R2-32 : powerlib/Elements/Series RLC Branch  LConnTagsString=__new0  RConnTagsString=__new0  BranchType=C  Resistance=1  Inductance=1e-3  SetiL0=off  InitialCurrent=0  Capacitance=Cbase/12.5  Setx0=off  InitialVoltage=0  Measurements=None
  Conn1 : PMIOPort  Port=1  Side=Right
  Conn2 : PMIOPort  Port=2  Side=Right
  Conn3 : PMIOPort  Port=3  Side=Right
  connections:
  R2-1/LConn1 -- Conn2/RConn1
  R2-2/LConn1 -- Conn3/RConn1
  R2-2/RConn1 -- R2-32/RConn1 -- Ground/LConn1 -- R2-1/RConn1
  R2-32/LConn1 -- Conn1/RConn1

== system ieee_6_bus_base_case_hydro_dominated/Subsystem2/B//8 ==
  Ground : powerlib/Elements/Ground  LConnTagsString=a
  R2-1 : powerlib/Elements/Series RLC Branch  LConnTagsString=__new0  RConnTagsString=__new0  BranchType=C  Resistance=1  Inductance=1e-3  SetiL0=off  InitialCurrent=0  Capacitance=Cbase/12.5  Setx0=off  InitialVoltage=0  Measurements=None
  R2-2 : powerlib/Elements/Series RLC Branch  LConnTagsString=__new0  RConnTagsString=__new0  BranchType=C  Resistance=1  Inductance=1e-3  SetiL0=off  InitialCurrent=0  Capacitance=Cbase/12.5  Setx0=off  InitialVoltage=0  Measurements=None
  R2-32 : powerlib/Elements/Series RLC Branch  LConnTagsString=__new0  RConnTagsString=__new0  BranchType=C  Resistance=1  Inductance=1e-3  SetiL0=off  InitialCurrent=0  Capacitance=Cbase/12.5  Setx0=off  InitialVoltage=0  Measurements=None
  Conn1 : PMIOPort  Port=1  Side=Right
  Conn2 : PMIOPort  Port=2  Side=Right
  Conn3 : PMIOPort  Port=3  Side=Right
  connections:
  R2-32/LConn1 -- Conn1/RConn1
  Ground/LConn1 -- R2-2/RConn1 -- R2-1/RConn1 -- R2-32/RConn1
  R2-2/LConn1 -- Conn3/RConn1
  R2-1/LConn1 -- Conn2/RConn1

== system ieee_6_bus_base_case_hydro_dominated/Subsystem3/B//11 ==
  Ground : powerlib/Elements/Ground  LConnTagsString=a
  R2-1 : powerlib/Elements/Series RLC Branch  LConnTagsString=__new0  RConnTagsString=__new0  BranchType=C  Resistance=1  Inductance=1e-3  SetiL0=off  InitialCurrent=0  Capacitance=(6*Cbase)/100  Setx0=off  InitialVoltage=0  Measurements=None
  R2-2 : powerlib/Elements/Series RLC Branch  LConnTagsString=__new0  RConnTagsString=__new0  BranchType=C  Resistance=1  Inductance=1e-3  SetiL0=off  InitialCurrent=0  Capacitance=(6*Cbase)/100  Setx0=off  InitialVoltage=0  Measurements=None
  R2-32 : powerlib/Elements/Series RLC Branch  LConnTagsString=__new0  RConnTagsString=__new0  BranchType=C  Resistance=1  Inductance=1e-3  SetiL0=off  InitialCurrent=0  Capacitance=(6*Cbase)/100  Setx0=off  InitialVoltage=0  Measurements=None
  Conn1 : PMIOPort  Port=1  Side=Right
  Conn2 : PMIOPort  Port=2  Side=Right
  Conn3 : PMIOPort  Port=3  Side=Right
  connections:
  R2-1/LConn1 -- Conn2/RConn1
  R2-2/LConn1 -- Conn3/RConn1
  R2-32/RConn1 -- R2-2/RConn1 -- R2-1/RConn1 -- Ground/LConn1
  R2-32/LConn1 -- Conn1/RConn1

== system ieee_6_bus_base_case_hydro_dominated/Subsystem3/B//12 ==
  Ground : powerlib/Elements/Ground  LConnTagsString=a
  R2-1 : powerlib/Elements/Series RLC Branch  LConnTagsString=__new0  RConnTagsString=__new0  BranchType=C  Resistance=1  Inductance=1e-3  SetiL0=off  InitialCurrent=0  Capacitance=(6*Cbase)/100  Setx0=off  InitialVoltage=0  Measurements=None
  R2-2 : powerlib/Elements/Series RLC Branch  LConnTagsString=__new0  RConnTagsString=__new0  BranchType=C  Resistance=1  Inductance=1e-3  SetiL0=off  InitialCurrent=0  Capacitance=(6*Cbase)/100  Setx0=off  InitialVoltage=0  Measurements=None
  R2-32 : powerlib/Elements/Series RLC Branch  LConnTagsString=__new0  RConnTagsString=__new0  BranchType=C  Resistance=1  Inductance=1e-3  SetiL0=off  InitialCurrent=0  Capacitance=(6*Cbase)/100  Setx0=off  InitialVoltage=0  Measurements=None
  Conn1 : PMIOPort  Port=1  Side=Right
  Conn2 : PMIOPort  Port=2  Side=Right
  Conn3 : PMIOPort  Port=3  Side=Right
  connections:
  R2-32/LConn1 -- Conn1/RConn1
  R2-2/RConn1 -- Ground/LConn1 -- R2-32/RConn1 -- R2-1/RConn1
  R2-2/LConn1 -- Conn3/RConn1
  R2-1/LConn1 -- Conn2/RConn1

== system ieee_6_bus_base_case_hydro_dominated/Subsystem4/B//19 ==
  Ground : powerlib/Elements/Ground  LConnTagsString=a
  R2-1 : powerlib/Elements/Series RLC Branch  LConnTagsString=__new0  RConnTagsString=__new0  BranchType=C  Resistance=1  Inductance=1e-3  SetiL0=off  InitialCurrent=0  Capacitance=Cbase/20  Setx0=off  InitialVoltage=0  Measurements=None
  R2-2 : powerlib/Elements/Series RLC Branch  LConnTagsString=__new0  RConnTagsString=__new0  BranchType=C  Resistance=1  Inductance=1e-3  SetiL0=off  InitialCurrent=0  Capacitance=Cbase/20  Setx0=off  InitialVoltage=0  Measurements=None
  R2-32 : powerlib/Elements/Series RLC Branch  LConnTagsString=__new0  RConnTagsString=__new0  BranchType=C  Resistance=1  Inductance=1e-3  SetiL0=off  InitialCurrent=0  Capacitance=Cbase/20  Setx0=off  InitialVoltage=0  Measurements=None
  Conn1 : PMIOPort  Port=1  Side=Right
  Conn2 : PMIOPort  Port=2  Side=Right
  Conn3 : PMIOPort  Port=3  Side=Right
  connections:
  R2-1/LConn1 -- Conn2/RConn1
  R2-2/LConn1 -- Conn3/RConn1
  R2-32/RConn1 -- R2-2/RConn1 -- R2-1/RConn1 -- Ground/LConn1
  R2-32/LConn1 -- Conn1/RConn1

== system ieee_6_bus_base_case_hydro_dominated/Subsystem4/B//20 ==
  Ground : powerlib/Elements/Ground  LConnTagsString=a
  R2-1 : powerlib/Elements/Series RLC Branch  LConnTagsString=__new0  RConnTagsString=__new0  BranchType=C  Resistance=1  Inductance=1e-3  SetiL0=off  InitialCurrent=0  Capacitance=Cbase/20  Setx0=off  InitialVoltage=0  Measurements=None
  R2-2 : powerlib/Elements/Series RLC Branch  LConnTagsString=__new0  RConnTagsString=__new0  BranchType=C  Resistance=1  Inductance=1e-3  SetiL0=off  InitialCurrent=0  Capacitance=Cbase/20  Setx0=off  InitialVoltage=0  Measurements=None
  R2-32 : powerlib/Elements/Series RLC Branch  LConnTagsString=__new0  RConnTagsString=__new0  BranchType=C  Resistance=1  Inductance=1e-3  SetiL0=off  InitialCurrent=0  Capacitance=Cbase/20  Setx0=off  InitialVoltage=0  Measurements=None
  Conn1 : PMIOPort  Port=1  Side=Right
  Conn2 : PMIOPort  Port=2  Side=Right
  Conn3 : PMIOPort  Port=3  Side=Right
  connections:
  R2-32/LConn1 -- Conn1/RConn1
  R2-2/RConn1 -- Ground/LConn1 -- R2-32/RConn1 -- R2-1/RConn1
  R2-2/LConn1 -- Conn3/RConn1
  R2-1/LConn1 -- Conn2/RConn1

== system ieee_6_bus_base_case_hydro_dominated/Subsystem5/B//10 ==
  Ground : powerlib/Elements/Ground  LConnTagsString=a
  R2-1 : powerlib/Elements/Series RLC Branch  LConnTagsString=__new0  RConnTagsString=__new0  BranchType=C  Resistance=1  Inductance=1e-3  SetiL0=off  InitialCurrent=0  Capacitance=Cbase/50  Setx0=off  InitialVoltage=0  Measurements=None
  R2-2 : powerlib/Elements/Series RLC Branch  LConnTagsString=__new0  RConnTagsString=__new0  BranchType=C  Resistance=1  Inductance=1e-3  SetiL0=off  InitialCurrent=0  Capacitance=Cbase/50  Setx0=off  InitialVoltage=0  Measurements=None
  R2-32 : powerlib/Elements/Series RLC Branch  LConnTagsString=__new0  RConnTagsString=__new0  BranchType=C  Resistance=1  Inductance=1e-3  SetiL0=off  InitialCurrent=0  Capacitance=Cbase/50  Setx0=off  InitialVoltage=0  Measurements=None
  Conn1 : PMIOPort  Port=1  Side=Right
  Conn2 : PMIOPort  Port=2  Side=Right
  Conn3 : PMIOPort  Port=3  Side=Right
  connections:
  R2-1/LConn1 -- Conn2/RConn1
  R2-2/LConn1 -- Conn3/RConn1
  R2-2/RConn1 -- R2-32/RConn1 -- Ground/LConn1 -- R2-1/RConn1
  R2-32/LConn1 -- Conn1/RConn1

== system ieee_6_bus_base_case_hydro_dominated/Subsystem5/B//9 ==
  Ground : powerlib/Elements/Ground  LConnTagsString=a
  R2-1 : powerlib/Elements/Series RLC Branch  LConnTagsString=__new0  RConnTagsString=__new0  BranchType=C  Resistance=1  Inductance=1e-3  SetiL0=off  InitialCurrent=0  Capacitance=Cbase/50  Setx0=off  InitialVoltage=0  Measurements=None
  R2-2 : powerlib/Elements/Series RLC Branch  LConnTagsString=__new0  RConnTagsString=__new0  BranchType=C  Resistance=1  Inductance=1e-3  SetiL0=off  InitialCurrent=0  Capacitance=Cbase/50  Setx0=off  InitialVoltage=0  Measurements=None
  R2-32 : powerlib/Elements/Series RLC Branch  LConnTagsString=__new0  RConnTagsString=__new0  BranchType=C  Resistance=1  Inductance=1e-3  SetiL0=off  InitialCurrent=0  Capacitance=Cbase/50  Setx0=off  InitialVoltage=0  Measurements=None
  Conn1 : PMIOPort  Port=1  Side=Right
  Conn2 : PMIOPort  Port=2  Side=Right
  Conn3 : PMIOPort  Port=3  Side=Right
  connections:
  R2-32/LConn1 -- Conn1/RConn1
  Ground/LConn1 -- R2-2/RConn1 -- R2-1/RConn1 -- R2-32/RConn1
  R2-2/LConn1 -- Conn3/RConn1
  R2-1/LConn1 -- Conn2/RConn1

== system ieee_6_bus_base_case_hydro_dominated/Subsystem6/B//16 ==
  C1 : powerlib/Elements/Series RLC Branch  LConnTagsString=__new0  RConnTagsString=__new0  BranchType=C  Resistance=1  Inductance=1e-3  SetiL0=off  InitialCurrent=0  Capacitance=Cbase/25  Setx0=off  InitialVoltage=0  Measurements=None
  C2 : powerlib/Elements/Series RLC Branch  LConnTagsString=__new0  RConnTagsString=__new0  BranchType=C  Resistance=1  Inductance=1e-3  SetiL0=off  InitialCurrent=0  Capacitance=Cbase/25  Setx0=off  InitialVoltage=0  Measurements=None
  C3 : powerlib/Elements/Series RLC Branch  LConnTagsString=__new0  RConnTagsString=__new0  BranchType=C  Resistance=1  Inductance=1e-3  SetiL0=off  InitialCurrent=0  Capacitance=Cbase/25  Setx0=off  InitialVoltage=0  Measurements=None
  Ground : powerlib/Elements/Ground  LConnTagsString=a
  Conn1 : PMIOPort  Port=1  Side=Right
  Conn2 : PMIOPort  Port=2  Side=Right
  Conn3 : PMIOPort  Port=3  Side=Right
  connections:
  C1/LConn1 -- Conn1/RConn1
  Ground/LConn1 -- C3/RConn1 -- C2/RConn1 -- C1/RConn1
  C3/LConn1 -- Conn3/RConn1
  C2/LConn1 -- Conn2/RConn1

== system ieee_6_bus_base_case_hydro_dominated/Subsystem6/B//18 ==
  C1 : powerlib/Elements/Series RLC Branch  LConnTagsString=__new0  RConnTagsString=__new0  BranchType=C  Resistance=1  Inductance=1e-3  SetiL0=off  InitialCurrent=0  Capacitance=Cbase/25  Setx0=off  InitialVoltage=0  Measurements=None
  C2 : powerlib/Elements/Series RLC Branch  LConnTagsString=__new0  RConnTagsString=__new0  BranchType=C  Resistance=1  Inductance=1e-3  SetiL0=off  InitialCurrent=0  Capacitance=Cbase/25  Setx0=off  InitialVoltage=0  Measurements=None
  C3 : powerlib/Elements/Series RLC Branch  LConnTagsString=__new0  RConnTagsString=__new0  BranchType=C  Resistance=1  Inductance=1e-3  SetiL0=off  InitialCurrent=0  Capacitance=Cbase/25  Setx0=off  InitialVoltage=0  Measurements=None
  Ground : powerlib/Elements/Ground  LConnTagsString=a
  Conn1 : PMIOPort  Port=1  Side=Right
  Conn2 : PMIOPort  Port=2  Side=Right
  Conn3 : PMIOPort  Port=3  Side=Right
  connections:
  C2/LConn1 -- Conn2/RConn1
  C3/LConn1 -- Conn3/RConn1
  C3/RConn1 -- C1/RConn1 -- Ground/LConn1 -- C2/RConn1
  C1/LConn1 -- Conn1/RConn1

== system ieee_6_bus_base_case_hydro_dominated/Subsystem7/B//13 ==
  Ground : powerlib/Elements/Ground  LConnTagsString=a
  R2-1 : powerlib/Elements/Series RLC Branch  LConnTagsString=__new0  RConnTagsString=__new0  BranchType=C  Resistance=1  Inductance=1e-3  SetiL0=off  InitialCurrent=0  Capacitance=Cbase/20  Setx0=off  InitialVoltage=0  Measurements=None
  R2-2 : powerlib/Elements/Series RLC Branch  LConnTagsString=__new0  RConnTagsString=__new0  BranchType=C  Resistance=1  Inductance=1e-3  SetiL0=off  InitialCurrent=0  Capacitance=Cbase/20  Setx0=off  InitialVoltage=0  Measurements=None
  R2-32 : powerlib/Elements/Series RLC Branch  LConnTagsString=__new0  RConnTagsString=__new0  BranchType=C  Resistance=1  Inductance=1e-3  SetiL0=off  InitialCurrent=0  Capacitance=Cbase/20  Setx0=off  InitialVoltage=0  Measurements=None
  Conn1 : PMIOPort  Port=1  Side=Right
  Conn2 : PMIOPort  Port=2  Side=Right
  Conn3 : PMIOPort  Port=3  Side=Right
  connections:
  R2-1/LConn1 -- Conn2/RConn1
  R2-2/LConn1 -- Conn3/RConn1
  R2-2/RConn1 -- R2-32/RConn1 -- Ground/LConn1 -- R2-1/RConn1
  R2-32/LConn1 -- Conn1/RConn1

== system ieee_6_bus_base_case_hydro_dominated/Subsystem7/B//14 ==
  Ground : powerlib/Elements/Ground  LConnTagsString=a
  R2-1 : powerlib/Elements/Series RLC Branch  LConnTagsString=__new0  RConnTagsString=__new0  BranchType=C  Resistance=1  Inductance=1e-3  SetiL0=off  InitialCurrent=0  Capacitance=Cbase/20  Setx0=off  InitialVoltage=0  Measurements=None
  R2-2 : powerlib/Elements/Series RLC Branch  LConnTagsString=__new0  RConnTagsString=__new0  BranchType=C  Resistance=1  Inductance=1e-3  SetiL0=off  InitialCurrent=0  Capacitance=Cbase/20  Setx0=off  InitialVoltage=0  Measurements=None
  R2-32 : powerlib/Elements/Series RLC Branch  LConnTagsString=__new0  RConnTagsString=__new0  BranchType=C  Resistance=1  Inductance=1e-3  SetiL0=off  InitialCurrent=0  Capacitance=Cbase/20  Setx0=off  InitialVoltage=0  Measurements=None
  Conn1 : PMIOPort  Port=1  Side=Right
  Conn2 : PMIOPort  Port=2  Side=Right
  Conn3 : PMIOPort  Port=3  Side=Right
  connections:
  R2-32/LConn1 -- Conn1/RConn1
  Ground/LConn1 -- R2-2/RConn1 -- R2-1/RConn1 -- R2-32/RConn1
  R2-2/LConn1 -- Conn3/RConn1
  R2-1/LConn1 -- Conn2/RConn1

== system ieee_6_bus_base_case_hydro_dominated/Subsystem8/B//21 ==
  C1 : powerlib/Elements/Series RLC Branch  LConnTagsString=__new0  RConnTagsString=__new0  BranchType=C  Resistance=1  Inductance=1e-3  SetiL0=off  InitialCurrent=0  Capacitance=(6*Cbase)/100  Setx0=off  InitialVoltage=0  Measurements=None
  C2 : powerlib/Elements/Series RLC Branch  LConnTagsString=__new0  RConnTagsString=__new0  BranchType=C  Resistance=1  Inductance=1e-3  SetiL0=off  InitialCurrent=0  Capacitance=(6*Cbase)/100  Setx0=off  InitialVoltage=0  Measurements=None
  C3 : powerlib/Elements/Series RLC Branch  LConnTagsString=__new0  RConnTagsString=__new0  BranchType=C  Resistance=1  Inductance=1e-3  SetiL0=off  InitialCurrent=0  Capacitance=(6*Cbase)/100  Setx0=off  InitialVoltage=0  Measurements=None
  Ground : powerlib/Elements/Ground  LConnTagsString=a
  Conn1 : PMIOPort  Port=1  Side=Right
  Conn2 : PMIOPort  Port=2  Side=Right
  Conn3 : PMIOPort  Port=3  Side=Right
  connections:
  C2/LConn1 -- Conn2/RConn1
  C3/LConn1 -- Conn3/RConn1
  C1/RConn1 -- C3/RConn1 -- C2/RConn1 -- Ground/LConn1
  C1/LConn1 -- Conn1/RConn1

== system ieee_6_bus_base_case_hydro_dominated/Subsystem8/B//22 ==
  C1 : powerlib/Elements/Series RLC Branch  LConnTagsString=__new0  RConnTagsString=__new0  BranchType=C  Resistance=1  Inductance=1e-3  SetiL0=off  InitialCurrent=0  Capacitance=(6*Cbase)/100  Setx0=off  InitialVoltage=0  Measurements=None
  C2 : powerlib/Elements/Series RLC Branch  LConnTagsString=__new0  RConnTagsString=__new0  BranchType=C  Resistance=1  Inductance=1e-3  SetiL0=off  InitialCurrent=0  Capacitance=(6*Cbase)/100  Setx0=off  InitialVoltage=0  Measurements=None
  C3 : powerlib/Elements/Series RLC Branch  LConnTagsString=__new0  RConnTagsString=__new0  BranchType=C  Resistance=1  Inductance=1e-3  SetiL0=off  InitialCurrent=0  Capacitance=(6*Cbase)/100  Setx0=off  InitialVoltage=0  Measurements=None
  Ground : powerlib/Elements/Ground  LConnTagsString=a
  Conn1 : PMIOPort  Port=1  Side=Right
  Conn2 : PMIOPort  Port=2  Side=Right
  Conn3 : PMIOPort  Port=3  Side=Right
  connections:
  C1/LConn1 -- Conn1/RConn1
  C3/RConn1 -- Ground/LConn1 -- C1/RConn1 -- C2/RConn1
  C3/LConn1 -- Conn3/RConn1
  C2/LConn1 -- Conn2/RConn1

== system ieee_6_bus_base_case_hydro_dominated/Subsystem9/B//15 ==
  Ground : powerlib/Elements/Ground  LConnTagsString=a
  R2-1 : powerlib/Elements/Series RLC Branch  LConnTagsString=__new0  RConnTagsString=__new0  BranchType=C  Resistance=1  Inductance=1e-3  SetiL0=off  InitialCurrent=0  Capacitance=(6*Cbase)/100  Setx0=off  InitialVoltage=0  Measurements=None
  R2-2 : powerlib/Elements/Series RLC Branch  LConnTagsString=__new0  RConnTagsString=__new0  BranchType=C  Resistance=1  Inductance=1e-3  SetiL0=off  InitialCurrent=0  Capacitance=(6*Cbase)/100  Setx0=off  InitialVoltage=0  Measurements=None
  R2-32 : powerlib/Elements/Series RLC Branch  LConnTagsString=__new0  RConnTagsString=__new0  BranchType=C  Resistance=1  Inductance=1e-3  SetiL0=off  InitialCurrent=0  Capacitance=(6*Cbase)/100  Setx0=off  InitialVoltage=0  Measurements=None
  Conn1 : PMIOPort  Port=1  Side=Right
  Conn2 : PMIOPort  Port=2  Side=Right
  Conn3 : PMIOPort  Port=3  Side=Right
  connections:
  R2-1/LConn1 -- Conn2/RConn1
  R2-2/LConn1 -- Conn3/RConn1
  R2-32/RConn1 -- R2-2/RConn1 -- R2-1/RConn1 -- Ground/LConn1
  R2-32/LConn1 -- Conn1/RConn1

== system ieee_6_bus_base_case_hydro_dominated/Subsystem9/B//6 ==
  Ground : powerlib/Elements/Ground  LConnTagsString=a
  R2-1 : powerlib/Elements/Series RLC Branch  LConnTagsString=__new0  RConnTagsString=__new0  BranchType=C  Resistance=1  Inductance=1e-3  SetiL0=off  InitialCurrent=0  Capacitance=(6*Cbase)/100  Setx0=off  InitialVoltage=0  Measurements=None
  R2-2 : powerlib/Elements/Series RLC Branch  LConnTagsString=__new0  RConnTagsString=__new0  BranchType=C  Resistance=1  Inductance=1e-3  SetiL0=off  InitialCurrent=0  Capacitance=(6*Cbase)/100  Setx0=off  InitialVoltage=0  Measurements=None
  R2-32 : powerlib/Elements/Series RLC Branch  LConnTagsString=__new0  RConnTagsString=__new0  BranchType=C  Resistance=1  Inductance=1e-3  SetiL0=off  InitialCurrent=0  Capacitance=(6*Cbase)/100  Setx0=off  InitialVoltage=0  Measurements=None
  Conn1 : PMIOPort  Port=1  Side=Right
  Conn2 : PMIOPort  Port=2  Side=Right
  Conn3 : PMIOPort  Port=3  Side=Right
  connections:
  R2-32/LConn1 -- Conn1/RConn1
  R2-2/RConn1 -- Ground/LConn1 -- R2-32/RConn1 -- R2-1/RConn1
  R2-2/LConn1 -- Conn3/RConn1
  R2-1/LConn1 -- Conn2/RConn1
